simulink library "QuaternionLibrary"  (R2023b)
settings: Solver=VariableStepAuto  StartTime=0.0  StopTime=10.0  RelTol=1e-3  EnableMultiTasking=on
settings Model: Creator=jeremie  LastModifiedBy=jerem
settings SolverCC: AlgebraicLoopSolver=TrustRegion
settings DataIOCC: LimitDataPoints=on
settings OptimizationCC: LifeSpan=inf
settings DebuggingCC: UnconnectedInputMsg=warning  UnconnectedOutputMsg=warning  UnconnectedLineMsg=warning  AllowSymbolicDim=off  SFUnexpectedBacktrackingDiag=warning  SFNoUnconditionalDefaultTransitionDiag=warning  SFExecutionAtInitializationDiag=none  ArithmeticOperatorsInVariantConditions=warning
settings ModelReferenceCC: EnableRefExpFcnMdlSchedulingChecks=on  PropagateSignalLabelsOutOfModel=off
settings SFSimCC: SimUseLocalCustomCode=off  CustomCodeUndefinedFunction=UseInterfaceOnly
settings RTWCC: RTWUseLocalCustomCode=off  DLArmComputeVersion=19.05
settings CodeAppCC: StateflowObjectComments=on
settings GRTTargetCC: TargetLangStandard=C89/C90 (ANSI)
settings ConfigComp: CovMetricSettings=dw  CovSaveCumulativeToWorkspaceVar=on  CovSaveSingleToWorkspaceVar=on  CovExternalEMLEnable=off

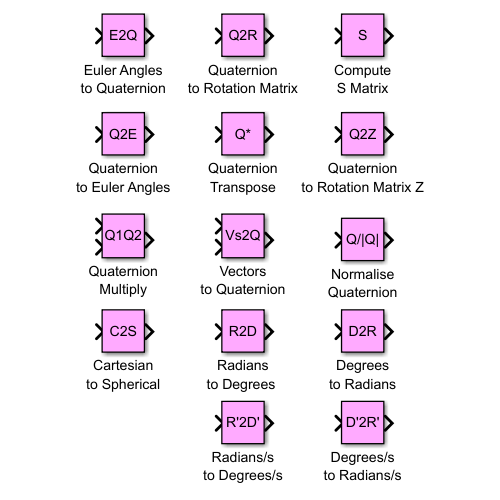
[thumbnail: Simulink's stored preview of the top-level diagram]
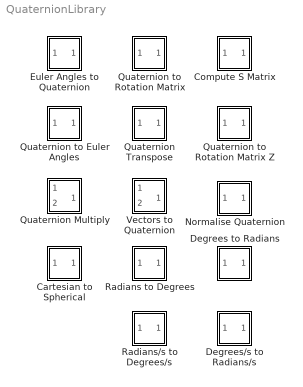
== system QuaternionLibrary ==
  Cartesian to Spherical : Subsystem
      mask help:
      | This block converts from cartesian to spherical coordinates in the form [azimuth; elevation; radius]
      |
      | When given a matrix input it outputs a matrix where each column corresponds to the spherical transformation of the corresponding column in the input vector.
      mask Display: disp('C2S')
  Compute S Matrix : Subsystem
      mask help: Convert an orientation quaternion to an orthogonal transformation matrix
      mask Help:
      | Convert a quaternion
      | [q1 q2 q3 q4]
      | to the S matrix used to compute angular acceleration and velocity quaternion
      | qDot = S * nuBody
      | 
      | qDDot = SDot * nuBody + S * nuBodyDot
      mask Display: disp('S')
  Degrees to Radians : Subsystem
      mask Display: disp('D2R')
  Degrees/s to Radians/s : Subsystem
      mask Display: disp('D''2R''')
  Euler Angles to Quaternion : Subsystem
      mask help: Convert vector of Euler angles to an orientation quaternion
      mask Help:
      | Convert vector of Euler angles
      | [roll, pitch, yaw]
      | to an orientation quaternion
      | [q1 q2 q3 q4]
      | where:
      | - q1 is the rotation in radians
      | - [q2 q3 q4] is the vector around which the rotation is performed)
      | 
      | Based on code from the PX4 firmware: https://github.com/PX4/Firmware
      mask Display: disp('E2Q')
  Normalise Quaternion : Subsystem
      mask help:
      | Normalise a quaternion
      |
      | Qhat = Q / |Q|
      mask Display: disp('Q/|Q|')
  Quaternion Multiply : Subsystem
      mask help:
      | Multiply two quaternions together
      |
      | Output = input1 (top) * input2 (bottom)
      mask Display: disp('Q1Q2')
  Quaternion Transpose : Subsystem
      mask help:
      | Find the transpose Q* of a quaternion Q
      |
      | [Q1* Q2* Q3* Q4*] = [Q1 -Q2 -Q3 -Q4]
      mask Display: disp('Q*')
  Quaternion to Euler Angles : Subsystem
      mask help: Convert an orientation quaternion to a vector of Euler angles
      mask Help:
      | Convert an orientation quaternion
      | [q1 q2 q3 q4]
      | where:
      | - q1 is the rotation in radians
      | - [q2 q3 q4] is the vector around which the rotation is performed)
      | to a vector of Euler angles
      | [roll, pitch, yaw]
      | Based on code from the PX4 firmware: https://github.com/PX4/Firmware
      mask Display: disp('Q2E')
  Quaternion to Rotation Matrix : Subsystem
      mask help: Convert an orientation quaternion to an orthogonal transformation matrix
      mask Help:
      | Convert an orientation quaternion
      | [q1 q2 q3 q4]
      | where:
      | - q1 is the rotation in radians
      | - [q2 q3 q4] is the vector around which the rotation is performed)
      | to an orthogonal transformation matrix
      | Based on code from the PX4 firmware: https://github.com/PX4/Firmware
      mask Display: disp('Q2R')
  Quaternion to Rotation Matrix Z : Subsystem
      mask help: Convert an orientation quaternion to an orthogonal transformation matrix
      mask Help:
      | Convert an orientation quaternion
      | [q1 q2 q3 q4]
      | where:
      | - q1 is the rotation in radians
      | - [q2 q3 q4] is the vector around which the rotation is performed)
      | to an orthogonal transformation matrix
      | Based on code from the PX4 firmware: https://github.com/PX4/Firmware
      mask Display: disp('Q2Z')
  "Radians to Degrees " : Subsystem
      mask Display: disp('R2D')
  Radians/s to Degrees/s : Subsystem
      mask Display: disp('R''2D''')
  Vectors to Quaternion : Subsystem
      mask help:
      | Multiply two quaternions together
      |
      | Output = input1 (top) * input2 (bottom)
      mask Display: disp('Vs2Q')

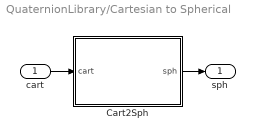
== system QuaternionLibrary/Cartesian to Spherical ==
  cart : Inport
  Cart2Sph : MATLAB Function  TreatAsAtomicUnit=on
  sph : Outport  VectorParamsAs1DForOutWhenUnconnected=off
  wires:
  Cart2Sph/1(sph) -> sph/1
  cart/1 -> Cart2Sph/1(cart)

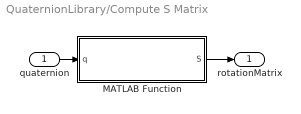
== system QuaternionLibrary/Compute S Matrix ==
  quaternion : Inport
  MATLAB Function : MATLAB Function  TreatAsAtomicUnit=on
  rotationMatrix : Outport  VectorParamsAs1DForOutWhenUnconnected=off
  wires:
  MATLAB Function/1(S) -> rotationMatrix/1
  quaternion/1 -> MATLAB Function/1(q)

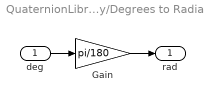
== system QuaternionLibrary/Degrees to Radians ==
  deg : Inport  Unit=deg
  Gain : Gain  Gain=pi/180
  rad : Outport  Unit=rad  VectorParamsAs1DForOutWhenUnconnected=off
  wires:
  Gain/1 -> rad/1
  deg/1 -> Gain/1

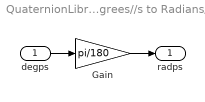
== system QuaternionLibrary/Degrees//s to Radians//s ==
  degps : Inport  Unit=deg/s
  Gain : Gain  Gain=pi/180
  radps : Outport  Unit=rad/s  VectorParamsAs1DForOutWhenUnconnected=off
  wires:
  degps/1 -> Gain/1
  Gain/1 -> radps/1

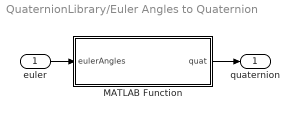
== system QuaternionLibrary/Euler Angles to Quaternion ==
  euler : Inport  Unit=rad
  MATLAB Function : MATLAB Function  TreatAsAtomicUnit=on
  quaternion : Outport  VectorParamsAs1DForOutWhenUnconnected=off
  wires:
  euler/1 -> MATLAB Function/1(eulerAngles)
  MATLAB Function/1(quat) -> quaternion/1

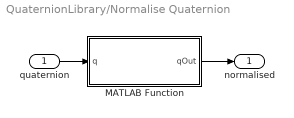
== system QuaternionLibrary/Normalise Quaternion ==
  quaternion : Inport
  MATLAB Function : MATLAB Function  TreatAsAtomicUnit=on
  normalised : Outport  VectorParamsAs1DForOutWhenUnconnected=off
  wires:
  MATLAB Function/1(qOut) -> normalised/1
  quaternion/1 -> MATLAB Function/1(q)

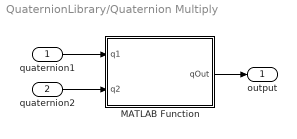
== system QuaternionLibrary/Quaternion Multiply ==
  quaternion1 : Inport
  quaternion2 : Inport  Port=2
  MATLAB Function : MATLAB Function  TreatAsAtomicUnit=on
  output : Outport  VectorParamsAs1DForOutWhenUnconnected=off
  wires:
  quaternion1/1 -> MATLAB Function/1(q1)
  MATLAB Function/1(qOut) -> output/1
  quaternion2/1 -> MATLAB Function/2(q2)

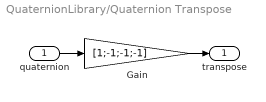
== system QuaternionLibrary/Quaternion Transpose ==
  quaternion : Inport
  Gain : Gain  Gain=[1;-1;-1;-1]
  transpose : Outport  VectorParamsAs1DForOutWhenUnconnected=off
  wires:
  quaternion/1 -> Gain/1
  Gain/1 -> transpose/1

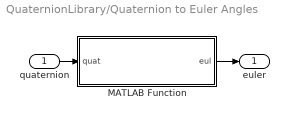
== system QuaternionLibrary/Quaternion to Euler Angles ==
  quaternion : Inport
  MATLAB Function : MATLAB Function  TreatAsAtomicUnit=on
  euler : Outport  Unit=rad  VectorParamsAs1DForOutWhenUnconnected=off
  wires:
  MATLAB Function/1(eul) -> euler/1
  quaternion/1 -> MATLAB Function/1(quat)

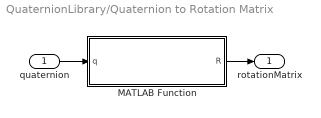
== system QuaternionLibrary/Quaternion to Rotation Matrix ==
  quaternion : Inport
  MATLAB Function : MATLAB Function  TreatAsAtomicUnit=on
  rotationMatrix : Outport  VectorParamsAs1DForOutWhenUnconnected=off
  wires:
  quaternion/1 -> MATLAB Function/1(q)
  MATLAB Function/1(R) -> rotationMatrix/1

== system QuaternionLibrary/Quaternion to Rotation Matrix Z ==
  quaternion : Inport  PortDimensions=4
  MATLAB Function : MATLAB Function  TreatAsAtomicUnit=on
  rotationMatrixZ : Outport  PortDimensions=3  VectorParamsAs1DForOutWhenUnconnected=off
  wires:
  MATLAB Function/1(dcmZ) -> rotationMatrixZ/1
  quaternion/1 -> MATLAB Function/1(quat)

== system QuaternionLibrary/Radians to Degrees  ==
  rad : Inport  Unit=rad
  Gain : Gain  Gain=180/pi
  deg : Outport  Unit=deg  VectorParamsAs1DForOutWhenUnconnected=off
  wires:
  rad/1 -> Gain/1
  Gain/1 -> deg/1

== system QuaternionLibrary/Radians//s to Degrees//s ==
  radps : Inport  Unit=rad/s
  Gain : Gain  Gain=180/pi
  degps : Outport  Unit=deg/s  VectorParamsAs1DForOutWhenUnconnected=off
  wires:
  Gain/1 -> degps/1
  radps/1 -> Gain/1

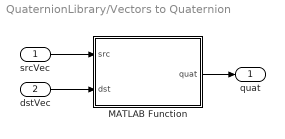
== system QuaternionLibrary/Vectors to Quaternion ==
  srcVec : Inport  PortDimensions=3
  dstVec : Inport  Port=2  PortDimensions=3
  MATLAB Function : MATLAB Function  TreatAsAtomicUnit=on
  quat : Outport  PortDimensions=4  VectorParamsAs1DForOutWhenUnconnected=off
  wires:
  dstVec/1 -> MATLAB Function/2(dst)
  MATLAB Function/1(quat) -> quat/1
  srcVec/1 -> MATLAB Function/1(src)

== matlab function QuaternionLibrary/Euler Angles to Quaternion/MATLAB Function ==
  data: eulerAngles input; quat output
function quat   = EulerToQuaternion( eulerAngles )
%EULERTOQUATERNION Convert Euler angles to a quaternion
%   Based on PX4 Firmware code: https://github.com/PX4/Firmware
%   Written by: J.X.J. Bannwarth
%   Last modified: 29/08/2016

    roll  = eulerAngles(1);
    pitch = eulerAngles(2);
    yaw   = eulerAngles(3);

    cosPhi_2   = cos(roll / 2.0);
    sinPhi_2   = sin(roll / 2.0);
    cosTheta_2 = cos(pitch / 2.0);
    sinTheta_2 = sin(pitch / 2.0);
    cosPsi_2   = cos(yaw / 2.0);
    sinPsi_2   = sin(yaw / 2.0);

    quat = [ cosPhi_2 .* cosTheta_2 .* cosPsi_2 + sinPhi_2 .* sinTheta_2 .* sinPsi_2;
             sinPhi_2 .* cosTheta_2 .* cosPsi_2 - cosPhi_2 .* sinTheta_2 .* sinPsi_2;
             cosPhi_2 .* sinTheta_2 .* cosPsi_2 + sinPhi_2 .* cosTheta_2 .* sinPsi_2;
             cosPhi_2 .* cosTheta_2 .* sinPsi_2 - sinPhi_2 .* sinTheta_2 .* cosPsi_2 ];

end

== matlab function QuaternionLibrary/Quaternion to Euler Angles/MATLAB Function ==
  data: quat input; eul output
function eul   = QuaternionToEuler( quat )
%QUATERNIONTOEULER Convert quaternion to euler angles
%   Based on PX4 Firmware code: https://github.com/PX4/Firmware
%   Written by:    J.X.J. Bannwarth, 2016/08/29
%   Last modified: J.X.J. Bannwarth, 2018/12/11

    eul = [ atan2(2.0 .* (quat(1) .* quat(2) + quat(3) .* quat(4)), ...
                1.0 - 2.0 .* (quat(2) .* quat(2) + quat(3) .* quat(3)));
	        asin(2.0 .* (quat(1) .* quat(3) - quat(4) .* quat(2)));
            atan2(2.0 .* (quat(1) .* quat(4) + quat(2) .* quat(3)), ...
                1.0 - 2.0 .* (quat(3) .* quat(3) + quat(4) .* quat(4))) ];
end

== matlab function QuaternionLibrary/Quaternion Multiply/MATLAB Function ==
  data: q1 input; qOut output; q2 input
function qOut   = QuatMult( q1, q2 )
%QUATMULT Multiply quaternion q1 by quaternion q2
%   Written by:    J.X.J. Bannwarth, 2017/03/28
%   Last modified: J.X.J. Bannwarth, 2018/12/11
    qOut = [ ...
        q1(1) * q2(1) - q1(2) * q2(2) - q1(3) * q2(3) - q1(4) * q2(4);
        q1(1) * q2(2) + q1(2) * q2(1) + q1(3) * q2(4) - q1(4) * q2(3);
        q1(1) * q2(3) - q1(2) * q2(4) + q1(3) * q2(1) + q1(4) * q2(2);
        q1(1) * q2(4) + q1(2) * q2(3) - q1(3) * q2(2) + q1(4) * q2(1) ...
        ];
end

== matlab function QuaternionLibrary/Normalise Quaternion/MATLAB Function ==
  data: q input; qOut output
function qOut = NormaliseQuat( q )
%NORMALISEQUAT Normalise quaternion
%   Based on PX4 Firmware code: https://github.com/PX4/Firmware
%   Written by:    J.X.J. Bannwarth, 2018/12/11
%   Last modified: J.X.J. Bannwarth, 2018/12/11

    qOut = zeros(4,1);
    normVal = sqrt( dot( q, q ) );
    if normVal ~= 0
        qOut = q ./ normVal;
    end
end

== matlab function QuaternionLibrary/Compute S Matrix/MATLAB Function ==
  data: q input; S output
function S = ComputeSMatrix(q)
%COMPUTESMATRIX Compute S Matrix
%   Written by:    J.X.J. Bannwarth, 2017/03/28
%   Last modified: J.X.J. Bannwarth, 2018/12/11
    S = zeros( 4, 3 );
    S(1,1) = -q(2) * 0.5;
    S(1,2) = -q(3) * 0.5;
    S(1,3) = -q(4) * 0.5;
    S(2,1) =  q(1) * 0.5;
    S(2,2) = -q(4) * 0.5;
    S(2,3) =  q(3) * 0.5;
    S(3,1) =  q(4) * 0.5;
    S(3,2) =  q(1) * 0.5;
    S(3,3) = -q(2) * 0.5;
    S(4,1) = -q(3) * 0.5;
    S(4,2) =  q(2) * 0.5;
    S(4,3) =  q(1) * 0.5;
end

== matlab function QuaternionLibrary/Quaternion to Rotation Matrix Z/MATLAB Function ==
  data: quat input; dcmZ output
function dcmZ = QuatToDcmZ( quat )
    %QUATTODCMZ Convert quaternion to corresponding body z-axis
    %	Last orthogonal unit basis vector
    %   == last column of the equivalent rotation matrix
    %   but calculated more efficiently than a full conversion
    %   Based on code from PX4 Firmware:
    %       https://github.com/PX4/Matrix/blob/master/matrix/Dcm.hpp
    %   Written:       J.X.J. Bannwarth, 2019/01/15
    %   Last modified: J.X.J. Bannwarth, 2019/01/15

    a = quat(1);
    b = quat(2);
    c = quat(3);
    d = quat(4);
    dcmZ = [ 2 * (a * c + b * d);
        2 * (c * d - a * b);
        a * a - b * b - c * c + d * d ];
end

== matlab function QuaternionLibrary/Vectors to Quaternion/MATLAB Function ==
  data: src input; quat output; dst input
function quat = VecsToQuat( src, dst )
    %VECSTOQUAT Quaternion from two vectors
    %   Generates shortest rotation from source to destination vector
    %   Based on code from PX4 Firmware:
    %       https://github.com/PX4/Matrix/blob/master/matrix/Quaternion.hpp
    %   Written:       J.X.J. Bannwarth, 2019/01/15
    %   Last modified: J.X.J. Bannwarth, 2019/01/15
    cr = cross(src, dst);
    dt = dot(src, dst);
    quat = zeros(4,1);
    locEps = 1e-5; % Don't use eps as it's a reserved variable in MATLAB
    if (norm(cr) < locEps && dt < 0)
        % Handle corner cases with 180 degree rotations
        % If the two vectors are parallel, cross product is zero
        % If they point opposite, the dot product is negative
        cr = abs(src);
        if (cr(1) < cr(2))
            if (cr(1) < cr(3))
                cr = [1; 0; 0];
            else
                cr = [0; 0; 1];
            end
        else
            if (cr(2) < cr(3))
                cr = [0; 1; 0];
            else
                cr = [0; 0; 1];
            end
        end
        quat(1) = 0;
        cr = cross(src, cr);
    else
        % Normal case, do half-way quaternion solution
        quat(1) = dt + sqrt( norm(src)^2 * norm(dst)^2 );
    end
    quat(2) = cr(1);
    quat(3) = cr(2);
    quat(4) = cr(3);
    quat = MulticopterAttitudeControl.normalize( quat );
end

== matlab function QuaternionLibrary/Cartesian to Spherical/Cart2Sph ==
  data: cart input; sph output
function sph = Cart2Sph( cart )
%#codegen
    x = cart(1,:); y = cart(2,:); z = cart(3,:);
    hypotxy = hypot( x, y );
    sph = [ atan2( y, x )      ; % azimuth 
            atan2( z, hypotxy ); % elevation
            hypot( hypotxy, z ); % radius
          ];
end

== matlab function QuaternionLibrary/Quaternion to Rotation Matrix/MATLAB Function ==
  data: q input; R output
function R = QuatToRot( q )
%QUATTOROT Convert quaternion to rotation matrix
%   Written by:    J.X.J. Bannwarth, 2017/03/27
%   Last modified: J.X.J. Bannwarth, 2018/12/11
    W = q(1);
    X = q(2);
    Y = q(3);
    Z = q(4);
    
    xx = X * X;
    xy = X * Y;
    xz = X * Z;
    xw = X * W;

    yy = Y * Y;
    yz = Y * Z;
    yw = Y * W;
    
    zz = Z * Z;
    zw = Z * W;

    m00 = 1 - 2 * ( yy + zz );
    m01 =     2 * ( xy - zw );
    m02 =     2 * ( xz + yw );

    m10 =     2 * ( xy + zw );
    m11 = 1 - 2 * ( xx + zz );
    m12 =     2 * ( yz - xw );

    m20 =     2 * ( xz - yw );
    m21 =     2 * ( yz + xw );
    m22 = 1 - 2 * ( xx + yy );
    
    R = [m00 m01 m02;
         m10 m11 m12;
         m20 m21 m22];   
end
